simulink model "paper_Exponential_Predefined_102"  (R2019a)
settings: Solver=ode4  StartTime=0.0  StopTime=40  FixedStep=0.001  RelTol=1e-3
libraries: simulink x6
(part 2 of 3)

== matlab function paper_Exponential_Predefined_102/yuding_zhishu1 ==
  data: t input; nta_1 output; t_f input; bta1 input; bta2 input; k1 input; k2 input; p1x input; p1y input; p1z input; p2x input; p2y input; p2z input; z2x input; z2y input; z2z input; nta_2 output; nta_3 output
function [nta_1,nta_2,nta_3] = yuding(t,t_f,bta1,bta2,k1,k2,p1x,p1y,p1z,p2x,p2y,p2z,z2x,z2y,z2z)
z2x=0;
z2y=0;
z2z=0;
if 0<t & t<t_f-0.01
[nta_1,nta_2,nta_3]=im_predefined(t,t_f,bta1,bta2,k1,k2,p1x,p1y,p1z,p2x,p2y,p2z,z2x,z2y,z2z);
else 
    nta_1=0;
    nta_2=0;
    nta_3=0;
    

%     tf=t_f;
%     deta_tf=4;     
%     if tf<=t & t<(tf+deta_tf-0.01)
%         [nta_1,nta_2,nta_3]=im_predefined(t,tf+deta_tf,bta1,bta2,k1,k2,p1x,p1y,p1z,p2x,p2y,p2z,z2x,z2y,z2z); 
%     else 
%         tf=tf+deta_tf;
%         [nta_1,nta_2,nta_3]=im_predefined(t,tf+deta_tf,bta1,bta2,k1,k2,p1x,p1y,p1z,p2x,p2y,p2z,z2x,z2y,z2z); 
%     end   
%     if tf<=t & t<(tf+deta_tf-0.01)
%         [nta_1,nta_2,nta_3]=im_predefined(t,tf+deta_tf,bta1,bta2,k1,k2,p1x,p1y,p1z,p2x,p2y,p2z,z2x,z2y,z2z); 
%     else
%         tf=tf+deta_tf;
%         [nta_1,nta_2,nta_3]=im_predefined(t,tf+deta_tf,bta1,bta2,k1,k2,p1x,p1y,p1z,p2x,p2y,p2z,z2x,z2y,z2z); 
%     end  
%     if tf<=t & t<(tf+deta_tf-0.01)
%         [nta_1,nta_2,nta_3]=im_predefined(t,tf+deta_tf,bta1,bta2,k1,k2,p1x,p1y,p1z,p2x,p2y,p2z,z2x,z2y,z2z); 
%     else
%         tf=tf+deta_tf;
%         [nta_1,nta_2,nta_3]=im_predefined(t,tf+deta_tf,bta1,bta2,k1,k2,p1x,p1y,p1z,p2x,p2y,p2z,z2x,z2y,z2z); 
%     end  
%     if tf<=t & t<(tf+deta_tf-0.01)
%         [nta_1,nta_2,nta_3]=im_predefined(t,tf+deta_tf,bta1,bta2,k1,k2,p1x,p1y,p1z,p2x,p2y,p2z,z2x,z2y,z2z); 
%     else
%         tf=tf+deta_tf;
%         [nta_1,nta_2,nta_3]=im_predefined(t,tf+deta_tf,bta1,bta2,k1,k2,p1x,p1y,p1z,p2x,p2y,p2z,z2x,z2y,z2z); 
%     end  
%     if tf<=t & t<(tf+deta_tf-0.01)
%         [nta_1,nta_2,nta_3]=im_predefined(t,tf+deta_tf,bta1,bta2,k1,k2,p1x,p1y,p1z,p2x,p2y,p2z,z2x,z2y,z2z); 
%     else
%         tf=tf+deta_tf;
%         [nta_1,nta_2,nta_3]=im_predefined(t,tf+deta_tf,bta1,bta2,k1,k2,p1x,p1y,p1z,p2x,p2y,p2z,z2x,z2y,z2z); 
%     end  
%     if tf<=t & t<(tf+deta_tf-0.01)
%         [nta_1,nta_2,nta_3]=im_predefined(t,tf+deta_tf,bta1,bta2,k1,k2,p1x,p1y,p1z,p2x,p2y,p2z,z2x,z2y,z2z); 
%     else
%         tf=tf+deta_tf;
%         [nta_1,nta_2,nta_3]=im_predefined(t,tf+deta_tf,bta1,bta2,k1,k2,p1x,p1y,p1z,p2x,p2y,p2z,z2x,z2y,z2z); 
%     end  
%     if tf<=t & t<(tf+deta_tf-0.01)
%         [nta_1,nta_2,nta_3]=im_predefined(t,tf+deta_tf,bta1,bta2,k1,k2,p1x,p1y,p1z,p2x,p2y,p2z,z2x,z2y,z2z); 
%     else
%         tf=tf+deta_tf;
%         [nta_1,nta_2,nta_3]=im_predefined(t,tf+deta_tf,bta1,bta2,k1,k2,p1x,p1y,p1z,p2x,p2y,p2z,z2x,z2y,z2z); 
%     end  
%     if tf<=t & t<(tf+deta_tf)
%         [nta_1,nta_2,nta_3]=im_predefined(t,tf+deta_tf,bta1,bta2,k1,k2,p1x,p1y,p1z,p2x,p2y,p2z,z2x,z2y,z2z); 
%     else
%         tf=tf+deta_tf;
%         [nta_1,nta_2,nta_3]=im_predefined(t,tf+deta_tf,bta1,bta2,k1,k2,p1x,p1y,p1z,p2x,p2y,p2z,z2x,z2y,z2z); 
%     end  
%     if tf<=t & t<(tf+deta_tf)
%         [nta_1,nta_2,nta_3]=im_predefined(t,tf+deta_tf,bta1,bta2,k1,k2,p1x,p1y,p1z,p2x,p2y,p2z,z2x,z2y,z2z); 
%     else
%         tf=tf+deta_tf;
%         [nta_1,nta_2,nta_3]=im_predefined(t,tf+deta_tf,bta1,bta2,k1,k2,p1x,p1y,p1z,p2x,p2y,p2z,z2x,z2y,z2z); 
%     end  
%     if tf<=t & t<(tf+deta_tf)
%         [nta_1,nta_2,nta_3]=im_predefined(t,tf+deta_tf,bta1,bta2,k1,k2,p1x,p1y,p1z,p2x,p2y,p2z,z2x,z2y,z2z); 
%     else
%         tf=tf+deta_tf;
%         [nta_1,nta_2,nta_3]=im_predefined(t,tf+deta_tf,bta1,bta2,k1,k2,p1x,p1y,p1z,p2x,p2y,p2z,z2x,z2y,z2z); 
%     end  
%     if tf<=t & t<(tf+deta_tf)
%         [nta_1,nta_2,nta_3]=im_predefined(t,tf+deta_tf,bta1,bta2,k1,k2,p1x,p1y,p1z,p2x,p2y,p2z,z2x,z2y,z2z); 
%     else
%         tf=tf+deta_tf;
%         [nta_1,nta_2,nta_3]=im_predefined(t,tf+deta_tf,bta1,bta2,k1,k2,p1x,p1y,p1z,p2x,p2y,p2z,z2x,z2y,z2z); 
%     end  
%     if tf<=t & t<(tf+deta_tf)
%         [nta_1,nta_2,nta_3]=im_predefined(t,tf+deta_tf,bta1,bta2,k1,k2,p1x,p1y,p1z,p2x,p2y,p2z,z2x,z2y,z2z); 
%     else
%         tf=tf+deta_tf;
%         [nta_1,nta_2,nta_3]=im_predefined(t,tf+deta_tf,bta1,bta2,k1,k2,p1x,p1y,p1z,p2x,p2y,p2z,z2x,z2y,z2z); 
%     end  
%     if tf<=t & t<(tf+deta_tf)
%         [nta_1,nta_2,nta_3]=im_predefined(t,tf+deta_tf,bta1,bta2,k1,k2,p1x,p1y,p1z,p2x,p2y,p2z,z2x,z2y,z2z); 
%     else
%         tf=tf+deta_tf;
%         [nta_1,nta_2,nta_3]=im_predefined(t,tf+deta_tf,bta1,bta2,k1,k2,p1x,p1y,p1z,p2x,p2y,p2z,z2x,z2y,z2z); 
%     end  
%     if tf<=t & t<(tf+deta_tf)
%         [nta_1,nta_2,nta_3]=im_predefined(t,tf+deta_tf,bta1,bta2,k1,k2,p1x,p1y,p1z,p2x,p2y,p2z,z2x,z2y,z2z); 
%     else
%         tf=tf+deta_tf;
%         [nta_1,nta_2,nta_3]=im_predefined(t,tf+deta_tf,bta1,bta2,k1,k2,p1x,p1y,p1z,p2x,p2y,p2z,z2x,z2y,z2z); 
%     end  
%     if tf<=t & t<(tf+deta_tf)
%         [nta_1,nta_2,nta_3]=im_predefined(t,tf+deta_tf,bta1,bta2,k1,k2,p1x,p1y,p1z,p2x,p2y,p2z,z2x,z2y,z2z); 
%     else
%         tf=tf+deta_tf;
%         [nta_1,nta_2,nta_3]=im_predefined(t,tf+deta_tf,bta1,bta2,k1,k2,p1x,p1y,p1z,p2x,p2y,p2z,z2x,z2y,z2z); 
%     end  
%     if tf<=t & t<(tf+deta_tf)
%         [nta_1,nta_2,nta_3]=im_predefined(t,tf+deta_tf,bta1,bta2,k1,k2,p1x,p1y,p1z,p2x,p2y,p2z,z2x,z2y,z2z); 
%     else
%         tf=tf+deta_tf;
%         [nta_1,nta_2,nta_3]=im_predefined(t,tf+deta_tf,bta1,bta2,k1,k2,p1x,p1y,p1z,p2x,p2y,p2z,z2x,z2y,z2z); 
%     end  
%     if tf<=t & t<(tf+deta_tf)
%         [nta_1,nta_2,nta_3]=im_predefined(t,tf+deta_tf,bta1,bta2,k1,k2,p1x,p1y,p1z,p2x,p2y,p2z,z2x,z2y,z2z); 
%     else
%         tf=tf+deta_tf;
%         [nta_1,nta_2,nta_3]=im_predefined(t,tf+deta_tf,bta1,bta2,k1,k2,p1x,p1y,p1z,p2x,p2y,p2z,z2x,z2y,z2z); 
%     end  
%     if tf<=t & t<(tf+deta_tf)
%         [nta_1,nta_2,nta_3]=im_predefined(t,tf+deta_tf,bta1,bta2,k1,k2,p1x,p1y,p1z,p2x,p2y,p2z,z2x,z2y,z2z); 
%     else
%         tf=tf+deta_tf;
%         [nta_1,nta_2,nta_3]=im_predefined(t,tf+deta_tf,bta1,bta2,k1,k2,p1x,p1y,p1z,p2x,p2y,p2z,z2x,z2y,z2z); 
%     end  
%     if tf<=t & t<(tf+deta_tf)
%         [nta_1,nta_2,nta_3]=im_predefined(t,tf+deta_tf,bta1,bta2,k1,k2,p1x,p1y,p1z,p2x,p2y,p2z,z2x,z2y,z2z); 
%     else
%         tf=tf+deta_tf;
%         [nta_1,nta_2,nta_3]=im_predefined(t,tf+deta_tf,bta1,bta2,k1,k2,p1x,p1y,p1z,p2x,p2y,p2z,z2x,z2y,z2z); 
%     end  
%     if tf<=t & t<(tf+deta_tf)
%         [nta_1,nta_2,nta_3]=im_predefined(t,tf+deta_tf,bta1,bta2,k1,k2,p1x,p1y,p1z,p2x,p2y,p2z,z2x,z2y,z2z); 
%     else
%         tf=tf+deta_tf;
%         [nta_1,nta_2,nta_3]=im_predefined(t,tf+deta_tf,bta1,bta2,k1,k2,p1x,p1y,p1z,p2x,p2y,p2z,z2x,z2y,z2z); 
%     end  
%     if tf<=t & t<(tf+deta_tf)
%         [nta_1,nta_2,nta_3]=im_predefined(t,tf+deta_tf,bta1,bta2,k1,k2,p1x,p1y,p1z,p2x,p2y,p2z,z2x,z2y,z2z); 
%     else
%         tf=tf+deta_tf;
%         [nta_1,nta_2,nta_3]=im_predefined(t,tf+deta_tf,bta1,bta2,k1,k2,p1x,p1y,p1z,p2x,p2y,p2z,z2x,z2y,z2z); 
%     end  
%     if tf<=t & t<(tf+deta_tf)
%         [nta_1,nta_2,nta_3]=im_predefined(t,tf+deta_tf,bta1,bta2,k1,k2,p1x,p1y,p1z,p2x,p2y,p2z,z2x,z2y,z2z); 
%     else
%         tf=tf+deta_tf;
%         [nta_1,nta_2,nta_3]=im_predefined(t,tf+deta_tf,bta1,bta2,k1,k2,p1x,p1y,p1z,p2x,p2y,p2z,z2x,z2y,z2z); 
%     end  
%     if tf<=t & t<(tf+deta_tf)
%         [nta_1,nta_2,nta_3]=im_predefined(t,tf+deta_tf,bta1,bta2,k1,k2,p1x,p1y,p1z,p2x,p2y,p2z,z2x,z2y,z2z); 
%     else
%         tf=tf+deta_tf;
%         [nta_1,nta_2,nta_3]=im_predefined(t,tf+deta_tf,bta1,bta2,k1,k2,p1x,p1y,p1z,p2x,p2y,p2z,z2x,z2y,z2z); 
%     end  
%     if tf<=t & t<(tf+deta_tf)
%         [nta_1,nta_2,nta_3]=im_predefined(t,tf+deta_tf,bta1,bta2,k1,k2,p1x,p1y,p1z,p2x,p2y,p2z,z2x,z2y,z2z); 
%     else
%         tf=tf+deta_tf;
%         [nta_1,nta_2,nta_3]=im_predefined(t,tf+deta_tf,bta1,bta2,k1,k2,p1x,p1y,p1z,p2x,p2y,p2z,z2x,z2y,z2z); 
%     end  
%     if tf<=t & t<(tf+deta_tf)
%         [nta_1,nta_2,nta_3]=im_predefined(t,tf+deta_tf,bta1,bta2,k1,k2,p1x,p1y,p1z,p2x,p2y,p2z,z2x,z2y,z2z); 
%     else
%         tf=tf+deta_tf;
%         [nta_1,nta_2,nta_3]=im_predefined(t,tf+deta_tf,bta1,bta2,k1,k2,p1x,p1y,p1z,p2x,p2y,p2z,z2x,z2y,z2z); 
%     end  
%     if tf<=t & t<(tf+deta_tf)
%         [nta_1,nta_2,nta_3]=im_predefined(t,tf+deta_tf,bta1,bta2,k1,k2,p1x,p1y,p1z,p2x,p2y,p2z,z2x,z2y,z2z); 
%     else
%         tf=tf+deta_tf;
%         [nta_1,nta_2,nta_3]=im_predefined(t,tf+deta_tf,bta1,bta2,k1,k2,p1x,p1y,p1z,p2x,p2y,p2z,z2x,z2y,z2z); 
%     end  
%         if tf<=t & t<(tf+deta_tf)
%         [nta_1,nta_2,nta_3]=im_predefined(t,tf+deta_tf,bta1,bta2,k1,k2,p1x,p1y,p1z,p2x,p2y,p2z,z2x,z2y,z2z); 
%     else
%         tf=tf+deta_tf;
%         [nta_1,nta_2,nta_3]=im_predefined(t,tf+deta_tf,bta1,bta2,k1,k2,p1x,p1y,p1z,p2x,p2y,p2z,z2x,z2y,z2z); 
%     end  
%     if tf<=t & t<(tf+deta_tf)
%         [nta_1,nta_2,nta_3]=im_predefined(t,tf+deta_tf,bta1,bta2,k1,k2,p1x,p1y,p1z,p2x,p2y,p2z,z2x,z2y,z2z); 
%     else
%         tf=tf+deta_tf;
%         [nta_1,nta_2,nta_3]=im_predefined(t,tf+deta_tf,bta1,bta2,k1,k2,p1x,p1y,p1z,p2x,p2y,p2z,z2x,z2y,z2z); 
%     end  
%         if tf<=t & t<(tf+deta_tf)
%         [nta_1,nta_2,nta_3]=im_predefined(t,tf+deta_tf,bta1,bta2,k1,k2,p1x,p1y,p1z,p2x,p2y,p2z,z2x,z2y,z2z); 
%     else
%         tf=tf+deta_tf;
%         [nta_1,nta_2,nta_3]=im_predefined(t,tf+deta_tf,bta1,bta2,k1,k2,p1x,p1y,p1z,p2x,p2y,p2z,z2x,z2y,z2z); 
%     end  
%     if tf<=t & t<(tf+deta_tf)
%         [nta_1,nta_2,nta_3]=im_predefined(t,tf+deta_tf,bta1,bta2,k1,k2,p1x,p1y,p1z,p2x,p2y,p2z,z2x,z2y,z2z); 
%     else
%         tf=tf+deta_tf;
%         [nta_1,nta_2,nta_3]=im_predefined(t,tf+deta_tf,bta1,bta2,k1,k2,p1x,p1y,p1z,p2x,p2y,p2z,z2x,z2y,z2z); 
%     end  
end    
end

== matlab function paper_Exponential_Predefined_102/MATLAB Function5 ==
  data: p1y input; p2y input; z0y input; dz0y output; dz1y output; dz2y output; z1y input; z2y input
function [dz0y,dz1y,dz2y] = FTDO(p1y,p2y,z0y,z1y,z2y)
r=[24 216 864];
r0=r(1);
r1=r(2);
r2=r(3);
v0=-r0*(abs(z0y-p1y))^(0.8)*sign(z0y-p1y)-r0*(abs(z0y-p1y))^(1.2)*sign(z0y-p1y)+z1y;
dz0y=v0+p2y;
v1=-r1*(abs(z0y-p1y))^(0.6)*sign(z0y-p1y)-r1*(abs(z0y-p1y))^(1.4)*sign(z0y-p1y)+z2y;
dz1y=v1;
dz2y =-r2*(abs(z0y-p1y))^(0.4)*sign(z0y-p1y)-r2*(abs(z0y-p1y))^(1.6)*sign(z0y-p1y);
end

== matlab function paper_Exponential_Predefined_102/MATLAB Function6 ==
  data: t input; dx output; dy output; dz output; delta input; v input; gamma input; psi input
function [dx,dy,dz] = disturbance(t,delta,v,gamma,psi)
fx=-0.0005*abs(v-36)*exp((0.4*v)^0.5)+0.2*sin(psi);
fy=-0.0004*abs(v-30)*exp((0.3*v)^0.5)+0.2*cos(psi);
fz=-0.004*v^(0.5)*sin(3*gamma);
% fx=0;
% fy=0;
% fz=0;
if 0<t && t<10
    wx = 1*sin(t)+delta;
else
    wx=0;
end
if 5<t && t<15
    wy = 2*sin(2*t)-cos(3*t)+delta;
else
    wy=0;
end
if 0<t && t<20
    wz = 0.5*sin(t)+delta;
else
    wz = 0;
end

dx=fx+wx;
dy=fy+wy;
dz=fz+wz;

end

== matlab function paper_Exponential_Predefined_102/MATLAB Function7 ==
  data: p1z input; p2z input; z0z input; dz0z output; dz1z output; dz2z output; z1z input; z2z input
function [dz0z,dz1z,dz2z] = FTDO(p1z,p2z,z0z,z1z,z2z)
r=[24 216 864];
r0=r(1);
r1=r(2);
r2=r(3);
v0=-r0*(abs(z0z-p1z))^(0.8)*sign(z0z-p1z)-r0*(abs(z0z-p1z))^(1.2)*sign(z0z-p1z)+z1z;
dz0z=v0+p2z;
v1=-r1*(abs(z0z-p1z))^(0.6)*sign(z0z-p1z)-r1*(abs(z0z-p1z))^(1.4)*sign(z0z-p1z)+z2z;
dz1z=v1;
dz2z =-r2*(abs(z0z-p1z))^(0.4)*sign(z0z-p1z)-r2*(abs(z0z-p1z))^(1.6)*sign(z0z-p1z);
end

== matlab function paper_Exponential_Predefined_102/MATLAB Function8 ==
  data: p1x input; p2x input; z0x input; dz0x output; dz1x output; dz2x output; z1x input; z2x input
function [dz0x,dz1x,dz2x] = FTDO(p1x,p2x,z0x,z1x,z2x)
r=[24 216 864];%parameters of FTDO
r0=r(1);
r1=r(2);
r2=r(3);
v0=-r0*(abs(z0x-p1x))^(0.8)*sign(z0x-p1x)-r0*(abs(z0x-p1x))^(1.2)*sign(z0x-p1x)+z1x;
dz0x=v0+p2x;
v1=-r1*(abs(z0x-p1x))^(0.6)*sign(z0x-p1x)-r1*(abs(z0x-p1x))^(1.4)*sign(z0x-p1x)+z2x;
dz1x=v1;
dz2x =-r2*(abs(z0x-p1x))^(0.4)*sign(z0x-p1x)-r2*(abs(z0x-p1x))^(1.6)*sign(z0x-p1x);
end

== matlab function paper_Exponential_Predefined_102/X_dot2 ==
  data: vr input; psi_r input; gamma_r input; psi input; gamma input; v input; s1 output; s2 output; s3 output; xr_dot output; yr_dot output; zr_dot output; wx input; wy input; wz input
function [s1,s2,s3,xr_dot,yr_dot,zr_dot] = fcn(vr,psi_r,gamma_r,psi,gamma,v,wx,wy,wz)
wx=0;
wy=0;
wz=0;
s1 = v*cos(psi)*cos(gamma)+wx;
s2 = v*sin(psi)*cos(gamma)+wy;
s3 = v*sin(gamma)+wz;
xr_dot = vr*cos(psi_r)*cos(gamma_r);
yr_dot = vr*sin(psi_r)*cos(gamma_r);
zr_dot = vr*sin(gamma_r);
end

== matlab function paper_Exponential_Predefined_102/control input 2 ==
  data: a_xr input; a_yr input; a_zr input; psi input; gamma input; u1_omiga_psi output; u2_omiga_gamma output; u3_a output; v input; nta_1 input; nta_2 input; nta_3 input
function [u1_omiga_psi,u2_omiga_gamma,u3_a] = fcn(a_xr,a_yr,a_zr,psi,gamma,v,nta_1,nta_2,nta_3)
A = [-a_xr;-a_yr;-a_zr];
B = [-v*sin(psi)*cos(gamma) -v*cos(psi)*sin(gamma) cos(psi)*cos(gamma); 
    v*cos(psi)*cos(gamma) -v*sin(psi)*sin(gamma) sin(psi)*cos(gamma);
    0                        v*cos(gamma)               sin(gamma)];
nta = [nta_1 ; nta_2;nta_3];
U = -inv(B)*(A - nta);
U11=U(1,1); 
U21=U(2,1);
U31=U(3,1);
% 

u1_omiga_psi = U11 ;
u2_omiga_gamma = U21;
u3_a =U31 ;





end

== matlab function paper_Exponential_Predefined_102/f,df2 ==
  data: dx input; x input; dy input; y input; dz input; z input; dxr input; xr input; dyr input; yr input; dzr input; zr input; p1x output; p1y output; p1z output; p2x output; p2y output; p2z output; wx input; wy input; wz input; s1 output; s2 output; s3 output
 function [p1x,p1y,p1z,p2x,p2y,p2z,s1,s2,s3] = fcn(dx,x,dy,y,dz,z,dxr,xr,dyr,yr,dzr,zr,wx,wy,wz)
wx=0;
wy=0;
wz=0;
p1x = x - xr;
p1y = y - yr;
p1z = z - zr;
s1 = dx - dxr ;
s2 = dy - dyr ;
s3 = dz - dzr ;
p2x = dx - dxr-wx ;
p2y = dy - dyr-wy ;
p2z = dz - dzr-wz ;
end

== matlab function paper_Exponential_Predefined_102/u_1a1 ==
  data: u input; u_1a output
function u_1a  = fcn(u)

u_max=1;

u_1a=u_max*erf((pi^(0.5)*u)/(2*u_max));


 end

== matlab function paper_Exponential_Predefined_102/u_2a2 ==
  data: u input; u_2a output
function u_2a  = fcn(u)

u_max=1;

u_2a=u_max*erf((pi^(0.5)*u)/(2*u_max));


 end

== matlab function paper_Exponential_Predefined_102/u_3a2 ==
  data: u input; u_3a output
function u_3a  = fcn(u)

u_max=10;
v_max=15;
% u_3a=u;
u_3a=u_max*erf((pi^(0.5)*u)/(2*u_max));
% q_v=erf((pi^(0.5)*(v-25))/(2*v_max));
% % u_3a=q_u*(1-abs(q_v));
% if v>=40 & u>0
%     u_3a=0;
% elseif v<=10 & u<0
%     u_3a=0;
% else
%     u_3a=u_max*erf((pi^(0.5)*u)/(2*u_max));
    
 end

== matlab function paper_Exponential_Predefined_102/yuding_zhishu2 ==
  data: t input; nta_1 output; t_f input; bta1 input; bta2 input; k1 input; k2 input; p1x input; p1y input; p1z input; p2x input; p2y input; p2z input; z2x input; z2y input; z2z input; nta_2 output; nta_3 output
function [nta_1,nta_2,nta_3] = yuding(t,t_f,bta1,bta2,k1,k2,p1x,p1y,p1z,p2x,p2y,p2z,z2x,z2y,z2z)
z2x=0;
z2y=0;
z2z=0;
if 0<t & t<t_f-0.01
[nta_1,nta_2,nta_3]=Exponential_predefined(t,t_f,bta1,bta2,k1,k2,p1x,p1y,p1z,p2x,p2y,p2z,z2x,z2y,z2z);
else 
% tf=[]
% for i=0:1:20
% tf(i)=t_f+i;
% if tf(i)<=t &t<(tf(i)+1)
% [nta_1,nta_2,nta_3]=Exponential_predefined_yuesu(t,tf(i)+1,bta1,bta2,k1,k2,p1x,p1y,p1z,p2x,p2y,p2z,z2x,z2y,z2z);
% end
% end
    tf=t_f;
    deta_tf=4;     
    if tf<=t & t<(tf+deta_tf-0.01)
        [nta_1,nta_2,nta_3]=Exponential_predefined(t,tf+deta_tf,bta1,bta2,k1,k2,p1x,p1y,p1z,p2x,p2y,p2z,z2x,z2y,z2z); 
    else 
        tf=tf+deta_tf;
        [nta_1,nta_2,nta_3]=Exponential_predefined(t,tf+deta_tf,bta1,bta2,k1,k2,p1x,p1y,p1z,p2x,p2y,p2z,z2x,z2y,z2z); 
    end   
    if tf<=t & t<(tf+deta_tf-0.01)
        [nta_1,nta_2,nta_3]=Exponential_predefined(t,tf+deta_tf,bta1,bta2,k1,k2,p1x,p1y,p1z,p2x,p2y,p2z,z2x,z2y,z2z); 
    else
        tf=tf+deta_tf;
        [nta_1,nta_2,nta_3]=Exponential_predefined(t,tf+deta_tf,bta1,bta2,k1,k2,p1x,p1y,p1z,p2x,p2y,p2z,z2x,z2y,z2z); 
    end  
    if tf<=t & t<(tf+deta_tf-0.01)
        [nta_1,nta_2,nta_3]=Exponential_predefined(t,tf+deta_tf,bta1,bta2,k1,k2,p1x,p1y,p1z,p2x,p2y,p2z,z2x,z2y,z2z); 
    else
        tf=tf+deta_tf;
        [nta_1,nta_2,nta_3]=Exponential_predefined(t,tf+deta_tf,bta1,bta2,k1,k2,p1x,p1y,p1z,p2x,p2y,p2z,z2x,z2y,z2z); 
    end  
    if tf<=t & t<(tf+deta_tf-0.01)
        [nta_1,nta_2,nta_3]=Exponential_predefined(t,tf+deta_tf,bta1,bta2,k1,k2,p1x,p1y,p1z,p2x,p2y,p2z,z2x,z2y,z2z); 
    else
        tf=tf+deta_tf;
        [nta_1,nta_2,nta_3]=Exponential_predefined(t,tf+deta_tf,bta1,bta2,k1,k2,p1x,p1y,p1z,p2x,p2y,p2z,z2x,z2y,z2z); 
    end  
    if tf<=t & t<(tf+deta_tf-0.01)
        [nta_1,nta_2,nta_3]=Exponential_predefined(t,tf+deta_tf,bta1,bta2,k1,k2,p1x,p1y,p1z,p2x,p2y,p2z,z2x,z2y,z2z); 
    else
        tf=tf+deta_tf;
        [nta_1,nta_2,nta_3]=Exponential_predefined(t,tf+deta_tf,bta1,bta2,k1,k2,p1x,p1y,p1z,p2x,p2y,p2z,z2x,z2y,z2z); 
    end  
    if tf<=t & t<(tf+deta_tf-0.01)
        [nta_1,nta_2,nta_3]=Exponential_predefined(t,tf+deta_tf,bta1,bta2,k1,k2,p1x,p1y,p1z,p2x,p2y,p2z,z2x,z2y,z2z); 
    else
        tf=tf+deta_tf;
        [nta_1,nta_2,nta_3]=Exponential_predefined(t,tf+deta_tf,bta1,bta2,k1,k2,p1x,p1y,p1z,p2x,p2y,p2z,z2x,z2y,z2z); 
    end  
    if tf<=t & t<(tf+deta_tf-0.01)
        [nta_1,nta_2,nta_3]=Exponential_predefined(t,tf+deta_tf,bta1,bta2,k1,k2,p1x,p1y,p1z,p2x,p2y,p2z,z2x,z2y,z2z); 
    else
        tf=tf+deta_tf;
        [nta_1,nta_2,nta_3]=Exponential_predefined(t,tf+deta_tf,bta1,bta2,k1,k2,p1x,p1y,p1z,p2x,p2y,p2z,z2x,z2y,z2z); 
    end  
    if tf<=t & t<(tf+deta_tf)
        [nta_1,nta_2,nta_3]=Exponential_predefined(t,tf+deta_tf,bta1,bta2,k1,k2,p1x,p1y,p1z,p2x,p2y,p2z,z2x,z2y,z2z); 
    else
        tf=tf+deta_tf;
        [nta_1,nta_2,nta_3]=Exponential_predefined(t,tf+deta_tf,bta1,bta2,k1,k2,p1x,p1y,p1z,p2x,p2y,p2z,z2x,z2y,z2z); 
    end  
    if tf<=t & t<(tf+deta_tf)
        [nta_1,nta_2,nta_3]=Exponential_predefined(t,tf+deta_tf,bta1,bta2,k1,k2,p1x,p1y,p1z,p2x,p2y,p2z,z2x,z2y,z2z); 
    else
        tf=tf+deta_tf;
        [nta_1,nta_2,nta_3]=Exponential_predefined(t,tf+deta_tf,bta1,bta2,k1,k2,p1x,p1y,p1z,p2x,p2y,p2z,z2x,z2y,z2z); 
    end  
    if tf<=t & t<(tf+deta_tf)
        [nta_1,nta_2,nta_3]=Exponential_predefined(t,tf+deta_tf,bta1,bta2,k1,k2,p1x,p1y,p1z,p2x,p2y,p2z,z2x,z2y,z2z); 
    else
        tf=tf+deta_tf;
        [nta_1,nta_2,nta_3]=Exponential_predefined(t,tf+deta_tf,bta1,bta2,k1,k2,p1x,p1y,p1z,p2x,p2y,p2z,z2x,z2y,z2z); 
    end  
    if tf<=t & t<(tf+deta_tf)
        [nta_1,nta_2,nta_3]=Exponential_predefined(t,tf+deta_tf,bta1,bta2,k1,k2,p1x,p1y,p1z,p2x,p2y,p2z,z2x,z2y,z2z); 
    else
        tf=tf+deta_tf;
        [nta_1,nta_2,nta_3]=Exponential_predefined(t,tf+deta_tf,bta1,bta2,k1,k2,p1x,p1y,p1z,p2x,p2y,p2z,z2x,z2y,z2z); 
    end  
    if tf<=t & t<(tf+deta_tf)
        [nta_1,nta_2,nta_3]=Exponential_predefined(t,tf+deta_tf,bta1,bta2,k1,k2,p1x,p1y,p1z,p2x,p2y,p2z,z2x,z2y,z2z); 
    else
        tf=tf+deta_tf;
        [nta_1,nta_2,nta_3]=Exponential_predefined(t,tf+deta_tf,bta1,bta2,k1,k2,p1x,p1y,p1z,p2x,p2y,p2z,z2x,z2y,z2z); 
    end  
    if tf<=t & t<(tf+deta_tf)
        [nta_1,nta_2,nta_3]=Exponential_predefined(t,tf+deta_tf,bta1,bta2,k1,k2,p1x,p1y,p1z,p2x,p2y,p2z,z2x,z2y,z2z); 
    else
        tf=tf+deta_tf;
        [nta_1,nta_2,nta_3]=Exponential_predefined(t,tf+deta_tf,bta1,bta2,k1,k2,p1x,p1y,p1z,p2x,p2y,p2z,z2x,z2y,z2z); 
    end  
    if tf<=t & t<(tf+deta_tf)
        [nta_1,nta_2,nta_3]=Exponential_predefined(t,tf+deta_tf,bta1,bta2,k1,k2,p1x,p1y,p1z,p2x,p2y,p2z,z2x,z2y,z2z); 
    else
        tf=tf+deta_tf;
        [nta_1,nta_2,nta_3]=Exponential_predefined(t,tf+deta_tf,bta1,bta2,k1,k2,p1x,p1y,p1z,p2x,p2y,p2z,z2x,z2y,z2z); 
    end  
    if tf<=t & t<(tf+deta_tf)
        [nta_1,nta_2,nta_3]=Exponential_predefined(t,tf+deta_tf,bta1,bta2,k1,k2,p1x,p1y,p1z,p2x,p2y,p2z,z2x,z2y,z2z); 
    else
        tf=tf+deta_tf;
        [nta_1,nta_2,nta_3]=Exponential_predefined(t,tf+deta_tf,bta1,bta2,k1,k2,p1x,p1y,p1z,p2x,p2y,p2z,z2x,z2y,z2z); 
    end  
    if tf<=t & t<(tf+deta_tf)
        [nta_1,nta_2,nta_3]=Exponential_predefined(t,tf+deta_tf,bta1,bta2,k1,k2,p1x,p1y,p1z,p2x,p2y,p2z,z2x,z2y,z2z); 
    else
        tf=tf+deta_tf;
        [nta_1,nta_2,nta_3]=Exponential_predefined(t,tf+deta_tf,bta1,bta2,k1,k2,p1x,p1y,p1z,p2x,p2y,p2z,z2x,z2y,z2z); 
    end  
    if tf<=t & t<(tf+deta_tf)
        [nta_1,nta_2,nta_3]=Exponential_predefined(t,tf+deta_tf,bta1,bta2,k1,k2,p1x,p1y,p1z,p2x,p2y,p2z,z2x,z2y,z2z); 
    else
        tf=tf+deta_tf;
        [nta_1,nta_2,nta_3]=Exponential_predefined(t,tf+deta_tf,bta1,bta2,k1,k2,p1x,p1y,p1z,p2x,p2y,p2z,z2x,z2y,z2z); 
    end  
    if tf<=t & t<(tf+deta_tf)
        [nta_1,nta_2,nta_3]=Exponential_predefined(t,tf+deta_tf,bta1,bta2,k1,k2,p1x,p1y,p1z,p2x,p2y,p2z,z2x,z2y,z2z); 
    else
        tf=tf+deta_tf;
        [nta_1,nta_2,nta_3]=Exponential_predefined(t,tf+deta_tf,bta1,bta2,k1,k2,p1x,p1y,p1z,p2x,p2y,p2z,z2x,z2y,z2z); 
    end  
    if tf<=t & t<(tf+deta_tf)
        [nta_1,nta_2,nta_3]=Exponential_predefined(t,tf+deta_tf,bta1,bta2,k1,k2,p1x,p1y,p1z,p2x,p2y,p2z,z2x,z2y,z2z); 
    else
        tf=tf+deta_tf;
        [nta_1,nta_2,nta_3]=Exponential_predefined(t,tf+deta_tf,bta1,bta2,k1,k2,p1x,p1y,p1z,p2x,p2y,p2z,z2x,z2y,z2z); 
    end  
    if tf<=t & t<(tf+deta_tf)
        [nta_1,nta_2,nta_3]=Exponential_predefined(t,tf+deta_tf,bta1,bta2,k1,k2,p1x,p1y,p1z,p2x,p2y,p2z,z2x,z2y,z2z); 
    else
        tf=tf+deta_tf;
        [nta_1,nta_2,nta_3]=Exponential_predefined(t,tf+deta_tf,bta1,bta2,k1,k2,p1x,p1y,p1z,p2x,p2y,p2z,z2x,z2y,z2z); 
    end  
    if tf<=t & t<(tf+deta_tf)
        [nta_1,nta_2,nta_3]=Exponential_predefined(t,tf+deta_tf,bta1,bta2,k1,k2,p1x,p1y,p1z,p2x,p2y,p2z,z2x,z2y,z2z); 
    else
        tf=tf+deta_tf;
        [nta_1,nta_2,nta_3]=Exponential_predefined(t,tf+deta_tf,bta1,bta2,k1,k2,p1x,p1y,p1z,p2x,p2y,p2z,z2x,z2y,z2z); 
    end  
    if tf<=t & t<(tf+deta_tf)
        [nta_1,nta_2,nta_3]=Exponential_predefined(t,tf+deta_tf,bta1,bta2,k1,k2,p1x,p1y,p1z,p2x,p2y,p2z,z2x,z2y,z2z); 
    else
        tf=tf+deta_tf;
        [nta_1,nta_2,nta_3]=Exponential_predefined(t,tf+deta_tf,bta1,bta2,k1,k2,p1x,p1y,p1z,p2x,p2y,p2z,z2x,z2y,z2z); 
    end  
    if tf<=t & t<(tf+deta_tf)
        [nta_1,nta_2,nta_3]=Exponential_predefined(t,tf+deta_tf,bta1,bta2,k1,k2,p1x,p1y,p1z,p2x,p2y,p2z,z2x,z2y,z2z); 
    else
        tf=tf+deta_tf;
        [nta_1,nta_2,nta_3]=Exponential_predefined(t,tf+deta_tf,bta1,bta2,k1,k2,p1x,p1y,p1z,p2x,p2y,p2z,z2x,z2y,z2z); 
    end  
    if tf<=t & t<(tf+deta_tf)
        [nta_1,nta_2,nta_3]=Exponential_predefined(t,tf+deta_tf,bta1,bta2,k1,k2,p1x,p1y,p1z,p2x,p2y,p2z,z2x,z2y,z2z); 
    else
        tf=tf+deta_tf;
        [nta_1,nta_2,nta_3]=Exponential_predefined(t,tf+deta_tf,bta1,bta2,k1,k2,p1x,p1y,p1z,p2x,p2y,p2z,z2x,z2y,z2z); 
    end  
    if tf<=t & t<(tf+deta_tf)
        [nta_1,nta_2,nta_3]=Exponential_predefined(t,tf+deta_tf,bta1,bta2,k1,k2,p1x,p1y,p1z,p2x,p2y,p2z,z2x,z2y,z2z); 
    else
        tf=tf+deta_tf;
        [nta_1,nta_2,nta_3]=Exponential_predefined(t,tf+deta_tf,bta1,bta2,k1,k2,p1x,p1y,p1z,p2x,p2y,p2z,z2x,z2y,z2z); 
    end  
    if tf<=t & t<(tf+deta_tf)
        [nta_1,nta_2,nta_3]=Exponential_predefined(t,tf+deta_tf,bta1,bta2,k1,k2,p1x,p1y,p1z,p2x,p2y,p2z,z2x,z2y,z2z); 
    else
        tf=tf+deta_tf;
        [nta_1,nta_2,nta_3]=Exponential_predefined(t,tf+deta_tf,bta1,bta2,k1,k2,p1x,p1y,p1z,p2x,p2y,p2z,z2x,z2y,z2z); 
    end  
        if tf<=t & t<(tf+deta_tf)
        [nta_1,nta_2,nta_3]=Exponential_predefined(t,tf+deta_tf,bta1,bta2,k1,k2,p1x,p1y,p1z,p2x,p2y,p2z,z2x,z2y,z2z); 
    else
        tf=tf+deta_tf;
        [nta_1,nta_2,nta_3]=Exponential_predefined(t,tf+deta_tf,bta1,bta2,k1,k2,p1x,p1y,p1z,p2x,p2y,p2z,z2x,z2y,z2z); 
    end  
    if tf<=t & t<(tf+deta_tf)
        [nta_1,nta_2,nta_3]=Exponential_predefined(t,tf+deta_tf,bta1,bta2,k1,k2,p1x,p1y,p1z,p2x,p2y,p2z,z2x,z2y,z2z); 
    else
        tf=tf+deta_tf;
        [nta_1,nta_2,nta_3]=Exponential_predefined(t,tf+deta_tf,bta1,bta2,k1,k2,p1x,p1y,p1z,p2x,p2y,p2z,z2x,z2y,z2z); 
    end  
        if tf<=t & t<(tf+deta_tf)
        [nta_1,nta_2,nta_3]=Exponential_predefined(t,tf+deta_tf,bta1,bta2,k1,k2,p1x,p1y,p1z,p2x,p2y,p2z,z2x,z2y,z2z); 
    else
        tf=tf+deta_tf;
        [nta_1,nta_2,nta_3]=Exponential_predefined(t,tf+deta_tf,bta1,bta2,k1,k2,p1x,p1y,p1z,p2x,p2y,p2z,z2x,z2y,z2z); 
    end  
    if tf<=t & t<(tf+deta_tf)
        [nta_1,nta_2,nta_3]=Exponential_predefined(t,tf+deta_tf,bta1,bta2,k1,k2,p1x,p1y,p1z,p2x,p2y,p2z,z2x,z2y,z2z); 
    else
        tf=tf+deta_tf;
        [nta_1,nta_2,nta_3]=Exponential_predefined(t,tf+deta_tf,bta1,bta2,k1,k2,p1x,p1y,p1z,p2x,p2y,p2z,z2x,z2y,z2z); 
    end  
end    
end

== matlab function paper_Exponential_Predefined_102/ a^r3 ==
  data: ar input; vr input; a_xr output; a_yr output; omiga_psi_r input; psi_r input; omiga_gamma_r input; a_zr output; gamma_r input
function [a_xr,a_yr,a_zr] = fcn(ar,vr,omiga_psi_r,psi_r,omiga_gamma_r,gamma_r)
a_xr = -vr*sin(psi_r)*cos(gamma_r)*omiga_psi_r-vr*cos(psi_r)*sin(gamma_r)*omiga_gamma_r+cos(psi_r)*cos(gamma_r)*ar;
a_yr = vr*cos(psi_r)*cos(gamma_r)*omiga_psi_r-vr*sin(psi_r)*sin(gamma_r)*omiga_gamma_r+ sin(psi_r)*cos(gamma_r)*ar;
a_zr = vr*cos(gamma_r)*omiga_gamma_r + sin(gamma_r)*ar;
end

== matlab function paper_Exponential_Predefined_102/MATLAB Function10 ==
  data: t input; dx output; dy output; dz output; delta input; v input; gamma input; psi input
function [dx,dy,dz] = disturbance(t,delta,v,gamma,psi)
fx=-0.0005*abs(v-36)*exp((0.4*v)^0.5)+0.2*sin(psi);
fy=-0.0004*abs(v-30)*exp((0.3*v)^0.5)+0.2*cos(psi);
fz=-0.004*v^(0.5)*sin(3*gamma);
% fx=0;
% fy=0;
% fz=0;
if 0<t && t<10
    wx = 1*sin(t)+delta;
else
    wx=0;
end
if 5<t && t<15
    wy = 2*sin(2*t)-cos(3*t)+delta;
else
    wy=0;
end
if 0<t && t<20
    wz = 0.5*sin(t)+delta;
else
    wz = 0;
end

dx=fx+wx;
dy=fy+wy;
dz=fz+wz;

end

== matlab function paper_Exponential_Predefined_102/MATLAB Function11 ==
  data: p1z input; p2z input; z0z input; dz0z output; dz1z output; dz2z output; z1z input; z2z input
function [dz0z,dz1z,dz2z] = FTDO(p1z,p2z,z0z,z1z,z2z)
r=[24 216 864];
r0=r(1);
r1=r(2);
r2=r(3);
v0=-r0*(abs(z0z-p1z))^(0.8)*sign(z0z-p1z)-r0*(abs(z0z-p1z))^(1.2)*sign(z0z-p1z)+z1z;
dz0z=v0+p2z;
v1=-r1*(abs(z0z-p1z))^(0.6)*sign(z0z-p1z)-r1*(abs(z0z-p1z))^(1.4)*sign(z0z-p1z)+z2z;
dz1z=v1;
dz2z =-r2*(abs(z0z-p1z))^(0.4)*sign(z0z-p1z)-r2*(abs(z0z-p1z))^(1.6)*sign(z0z-p1z);
end

== matlab function paper_Exponential_Predefined_102/MATLAB Function12 ==
  data: p1x input; p2x input; z0x input; dz0x output; dz1x output; dz2x output; z1x input; z2x input
function [dz0x,dz1x,dz2x] = FTDO(p1x,p2x,z0x,z1x,z2x)
r=[24 216 864];
r0=r(1);
r1=r(2);
r2=r(3);
v0=-r0*(abs(z0x-p1x))^(0.8)*sign(z0x-p1x)-r0*(abs(z0x-p1x))^(1.2)*sign(z0x-p1x)+z1x;
dz0x=v0+p2x;
% dz0x=v0;
v1=-r1*(abs(z0x-p1x))^(0.6)*sign(z0x-p1x)-r1*(abs(z0x-p1x))^(1.4)*sign(z0x-p1x)+z2x;
dz1x=v1;
dz2x =-r2*(abs(z0x-p1x))^(0.4)*sign(z0x-p1x)-r2*(abs(z0x-p1x))^(1.6)*sign(z0x-p1x);
end

== matlab function paper_Exponential_Predefined_102/MATLAB Function9 ==
  data: p1y input; p2y input; z0y input; dz0y output; dz1y output; dz2y output; z1y input; z2y input
function [dz0y,dz1y,dz2y] = FTDO(p1y,p2y,z0y,z1y,z2y)
r=[24 216 864];
r0=r(1);
r1=r(2);
r2=r(3);
v0=-r0*(abs(z0y-p1y))^(0.8)*sign(z0y-p1y)-r0*(abs(z0y-p1y))^(1.2)*sign(z0y-p1y)+z1y;
dz0y=v0+p2y;
v1=-r1*(abs(z0y-p1y))^(0.6)*sign(z0y-p1y)-r1*(abs(z0y-p1y))^(1.4)*sign(z0y-p1y)+z2y;
dz1y=v1;
dz2y =-r2*(abs(z0y-p1y))^(0.4)*sign(z0y-p1y)-r2*(abs(z0y-p1y))^(1.6)*sign(z0y-p1y);
end

== matlab function paper_Exponential_Predefined_102/X_dot3 ==
  data: vr input; psi_r input; gamma_r input; psi input; gamma input; v input; s1 output; s2 output; s3 output; xr_dot output; yr_dot output; zr_dot output; wx input; wy input; wz input
function [s1,s2,s3,xr_dot,yr_dot,zr_dot] = fcn(vr,psi_r,gamma_r,psi,gamma,v,wx,wy,wz)
% wx=0;
% wy=0;
% wz=0;
s1 = v*cos(psi)*cos(gamma)+wx;
s2 = v*sin(psi)*cos(gamma)+wy;
s3 = v*sin(gamma)+wz;
xr_dot = vr*cos(psi_r)*cos(gamma_r);
yr_dot = vr*sin(psi_r)*cos(gamma_r);
zr_dot = vr*sin(gamma_r);
end

== matlab function paper_Exponential_Predefined_102/control input 3 ==
  data: a_xr input; a_yr input; a_zr input; psi input; gamma input; u1_omiga_psi output; u2_omiga_gamma output; u3_a output; v input; nta_1 input; nta_2 input; nta_3 input
function [u1_omiga_psi,u2_omiga_gamma,u3_a] = fcn(a_xr,a_yr,a_zr,psi,gamma,v,nta_1,nta_2,nta_3)
A = [-a_xr;-a_yr;-a_zr];
B = [-v*sin(psi)*cos(gamma) -v*cos(psi)*sin(gamma) cos(psi)*cos(gamma); 
    v*cos(psi)*cos(gamma) -v*sin(psi)*sin(gamma) sin(psi)*cos(gamma);
    0                        v*cos(gamma)               sin(gamma)];
nta = [nta_1 ; nta_2;nta_3];
U = -inv(B)*(A - nta);
U11=U(1,1); 
U21=U(2,1);
U31=U(3,1);
% 

u1_omiga_psi = U11 ;
u2_omiga_gamma = U21;
u3_a =U31 ;
%%添加约束





end

== matlab function paper_Exponential_Predefined_102/f,df3 ==
  data: dx input; x input; dy input; y input; dz input; z input; dxr input; xr input; dyr input; yr input; dzr input; zr input; p1x output; p1y output; p1z output; p2x output; p2y output; p2z output; wx input; wy input; wz input; s1 output; s2 output; s3 output
 function [p1x,p1y,p1z,p2x,p2y,p2z,s1,s2,s3] = fcn(dx,x,dy,y,dz,z,dxr,xr,dyr,yr,dzr,zr,wx,wy,wz)
% wx=0;
% wy=0;
% wz=0;
p1x = x - xr;
p1y = y - yr;
p1z = z - zr;
s1 = dx - dxr ;
s2 = dy - dyr ;
s3 = dz - dzr ;
p2x = dx - dxr-wx ;
p2y = dy - dyr-wy ;
p2z = dz - dzr-wz ;
end

== matlab function paper_Exponential_Predefined_102/u_1a3 ==
  data: u input; u_1a output
function u_1a  = fcn(u)

u_max=1.6;

u_1a=u_max*erf((pi^(0.5)*u)/(2*u_max));


 end

== matlab function paper_Exponential_Predefined_102/u_2a3 ==
  data: u input; u_2a output
function u_2a  = fcn(u)

u_max=1.6;

u_2a=u_max*erf((pi^(0.5)*u)/(2*u_max));


 end

== matlab function paper_Exponential_Predefined_102/u_3a3 ==
  data: u input; u_3a output
function u_3a  = fcn(u)

u_max=17;
v_max=15;
% u_3a=u;
u_3a=u_max*erf((pi^(0.5)*u)/(2*u_max));
% q_v=erf((pi^(0.5)*(v-25))/(2*v_max));
% % u_3a=q_u*(1-abs(q_v));
% if v>=40 & u>0
%     u_3a=0;
% elseif v<=10 & u<0
%     u_3a=0;
% else
%     u_3a=u_max*erf((pi^(0.5)*u)/(2*u_max));
    
 end

== matlab function paper_Exponential_Predefined_102/yuding_zhishu3 ==
  data: t input; nta_1 output; t_f input; bta1 input; bta2 input; k1 input; k2 input; p1x input; p1y input; p1z input; p2x input; p2y input; p2z input; z2x input; z2y input; z2z input; nta_2 output; nta_3 output
function [nta_1,nta_2,nta_3] = predefined(t,t_f,bta1,bta2,k1,k2,p1x,p1y,p1z,p2x,p2y,p2z,z2x,z2y,z2z)
% z2x=0;
% z2y=0;
% z2z=0;
if 0<t & t<t_f-0.01
[nta_1,nta_2,nta_3]=im_predefined(t,t_f,bta1,bta2,k1,k2,p1x,p1y,p1z,p2x,p2y,p2z,z2x,z2y,z2z);
else 
%     nta_1=0;
%     nta_2=0;       
%     nta_3=0;
    

    tf=t_f;
    deta_tf=10;     
    if tf<=t & t<(tf+deta_tf-0.01)
        [nta_1,nta_2,nta_3]=im_predefined(t,tf+deta_tf,bta1,bta2,k1,k2,p1x,p1y,p1z,p2x,p2y,p2z,z2x,z2y,z2z); 
    else 
        tf=tf+deta_tf;
        [nta_1,nta_2,nta_3]=im_predefined(t,tf+deta_tf,bta1,bta2,k1,k2,p1x,p1y,p1z,p2x,p2y,p2z,z2x,z2y,z2z); 
    end   
    if tf<=t & t<(tf+deta_tf-0.01)
        [nta_1,nta_2,nta_3]=im_predefined(t,tf+deta_tf,bta1,bta2,k1,k2,p1x,p1y,p1z,p2x,p2y,p2z,z2x,z2y,z2z); 
    else
        tf=tf+deta_tf;
        [nta_1,nta_2,nta_3]=im_predefined(t,tf+deta_tf,bta1,bta2,k1,k2,p1x,p1y,p1z,p2x,p2y,p2z,z2x,z2y,z2z); 
    end  
    if tf<=t & t<(tf+deta_tf-0.01)
        [nta_1,nta_2,nta_3]=im_predefined(t,tf+deta_tf,bta1,bta2,k1,k2,p1x,p1y,p1z,p2x,p2y,p2z,z2x,z2y,z2z); 
    else
        tf=tf+deta_tf;
        [nta_1,nta_2,nta_3]=im_predefined(t,tf+deta_tf,bta1,bta2,k1,k2,p1x,p1y,p1z,p2x,p2y,p2z,z2x,z2y,z2z); 
    end  
    if tf<=t & t<(tf+deta_tf-0.01)
        [nta_1,nta_2,nta_3]=im_predefined(t,tf+deta_tf,bta1,bta2,k1,k2,p1x,p1y,p1z,p2x,p2y,p2z,z2x,z2y,z2z); 
    else
        tf=tf+deta_tf;
        [nta_1,nta_2,nta_3]=im_predefined(t,tf+deta_tf,bta1,bta2,k1,k2,p1x,p1y,p1z,p2x,p2y,p2z,z2x,z2y,z2z); 
    end  
    if tf<=t & t<(tf+deta_tf-0.01)
        [nta_1,nta_2,nta_3]=im_predefined(t,tf+deta_tf,bta1,bta2,k1,k2,p1x,p1y,p1z,p2x,p2y,p2z,z2x,z2y,z2z); 
    else
        tf=tf+deta_tf;
        [nta_1,nta_2,nta_3]=im_predefined(t,tf+deta_tf,bta1,bta2,k1,k2,p1x,p1y,p1z,p2x,p2y,p2z,z2x,z2y,z2z); 
    end  
    if tf<=t & t<(tf+deta_tf-0.01)
        [nta_1,nta_2,nta_3]=im_predefined(t,tf+deta_tf,bta1,bta2,k1,k2,p1x,p1y,p1z,p2x,p2y,p2z,z2x,z2y,z2z); 
    else
        tf=tf+deta_tf;
        [nta_1,nta_2,nta_3]=im_predefined(t,tf+deta_tf,bta1,bta2,k1,k2,p1x,p1y,p1z,p2x,p2y,p2z,z2x,z2y,z2z); 
    end  
    if tf<=t & t<(tf+deta_tf-0.01)
        [nta_1,nta_2,nta_3]=im_predefined(t,tf+deta_tf,bta1,bta2,k1,k2,p1x,p1y,p1z,p2x,p2y,p2z,z2x,z2y,z2z); 
    else
        tf=tf+deta_tf;
        [nta_1,nta_2,nta_3]=im_predefined(t,tf+deta_tf,bta1,bta2,k1,k2,p1x,p1y,p1z,p2x,p2y,p2z,z2x,z2y,z2z); 
    end  
    if tf<=t & t<(tf+deta_tf)
        [nta_1,nta_2,nta_3]=im_predefined(t,tf+deta_tf,bta1,bta2,k1,k2,p1x,p1y,p1z,p2x,p2y,p2z,z2x,z2y,z2z); 
    else
        tf=tf+deta_tf;
        [nta_1,nta_2,nta_3]=im_predefined(t,tf+deta_tf,bta1,bta2,k1,k2,p1x,p1y,p1z,p2x,p2y,p2z,z2x,z2y,z2z); 
    end  
    if tf<=t & t<(tf+deta_tf)
        [nta_1,nta_2,nta_3]=im_predefined(t,tf+deta_tf,bta1,bta2,k1,k2,p1x,p1y,p1z,p2x,p2y,p2z,z2x,z2y,z2z); 
    else
        tf=tf+deta_tf;
        [nta_1,nta_2,nta_3]=im_predefined(t,tf+deta_tf,bta1,bta2,k1,k2,p1x,p1y,p1z,p2x,p2y,p2z,z2x,z2y,z2z); 
    end  
    if tf<=t & t<(tf+deta_tf)
        [nta_1,nta_2,nta_3]=im_predefined(t,tf+deta_tf,bta1,bta2,k1,k2,p1x,p1y,p1z,p2x,p2y,p2z,z2x,z2y,z2z); 
    else
        tf=tf+deta_tf;
        [nta_1,nta_2,nta_3]=im_predefined(t,tf+deta_tf,bta1,bta2,k1,k2,p1x,p1y,p1z,p2x,p2y,p2z,z2x,z2y,z2z); 
    end  
    if tf<=t & t<(tf+deta_tf)
        [nta_1,nta_2,nta_3]=im_predefined(t,tf+deta_tf,bta1,bta2,k1,k2,p1x,p1y,p1z,p2x,p2y,p2z,z2x,z2y,z2z); 
    else
        tf=tf+deta_tf;
        [nta_1,nta_2,nta_3]=im_predefined(t,tf+deta_tf,bta1,bta2,k1,k2,p1x,p1y,p1z,p2x,p2y,p2z,z2x,z2y,z2z); 
    end  
    if tf<=t & t<(tf+deta_tf)
        [nta_1,nta_2,nta_3]=im_predefined(t,tf+deta_tf,bta1,bta2,k1,k2,p1x,p1y,p1z,p2x,p2y,p2z,z2x,z2y,z2z); 
    else
        tf=tf+deta_tf;
        [nta_1,nta_2,nta_3]=im_predefined(t,tf+deta_tf,bta1,bta2,k1,k2,p1x,p1y,p1z,p2x,p2y,p2z,z2x,z2y,z2z); 
    end  
    if tf<=t & t<(tf+deta_tf)
        [nta_1,nta_2,nta_3]=im_predefined(t,tf+deta_tf,bta1,bta2,k1,k2,p1x,p1y,p1z,p2x,p2y,p2z,z2x,z2y,z2z); 
    else
        tf=tf+deta_tf;
        [nta_1,nta_2,nta_3]=im_predefined(t,tf+deta_tf,bta1,bta2,k1,k2,p1x,p1y,p1z,p2x,p2y,p2z,z2x,z2y,z2z); 
    end  
    if tf<=t & t<(tf+deta_tf)
        [nta_1,nta_2,nta_3]=im_predefined(t,tf+deta_tf,bta1,bta2,k1,k2,p1x,p1y,p1z,p2x,p2y,p2z,z2x,z2y,z2z); 
    else
        tf=tf+deta_tf;
        [nta_1,nta_2,nta_3]=im_predefined(t,tf+deta_tf,bta1,bta2,k1,k2,p1x,p1y,p1z,p2x,p2y,p2z,z2x,z2y,z2z); 
    end  
    if tf<=t & t<(tf+deta_tf)
        [nta_1,nta_2,nta_3]=im_predefined(t,tf+deta_tf,bta1,bta2,k1,k2,p1x,p1y,p1z,p2x,p2y,p2z,z2x,z2y,z2z); 
    else
        tf=tf+deta_tf;
        [nta_1,nta_2,nta_3]=im_predefined(t,tf+deta_tf,bta1,bta2,k1,k2,p1x,p1y,p1z,p2x,p2y,p2z,z2x,z2y,z2z); 
    end  
    if tf<=t & t<(tf+deta_tf)
        [nta_1,nta_2,nta_3]=im_predefined(t,tf+deta_tf,bta1,bta2,k1,k2,p1x,p1y,p1z,p2x,p2y,p2z,z2x,z2y,z2z); 
    else
        tf=tf+deta_tf;
        [nta_1,nta_2,nta_3]=im_predefined(t,tf+deta_tf,bta1,bta2,k1,k2,p1x,p1y,p1z,p2x,p2y,p2z,z2x,z2y,z2z); 
    end  
    if tf<=t & t<(tf+deta_tf)
        [nta_1,nta_2,nta_3]=im_predefined(t,tf+deta_tf,bta1,bta2,k1,k2,p1x,p1y,p1z,p2x,p2y,p2z,z2x,z2y,z2z); 
    else
        tf=tf+deta_tf;
        [nta_1,nta_2,nta_3]=im_predefined(t,tf+deta_tf,bta1,bta2,k1,k2,p1x,p1y,p1z,p2x,p2y,p2z,z2x,z2y,z2z); 
    end  
    if tf<=t & t<(tf+deta_tf)
        [nta_1,nta_2,nta_3]=im_predefined(t,tf+deta_tf,bta1,bta2,k1,k2,p1x,p1y,p1z,p2x,p2y,p2z,z2x,z2y,z2z); 
    else
        tf=tf+deta_tf;
        [nta_1,nta_2,nta_3]=im_predefined(t,tf+deta_tf,bta1,bta2,k1,k2,p1x,p1y,p1z,p2x,p2y,p2z,z2x,z2y,z2z); 
    end  
    if tf<=t & t<(tf+deta_tf)
        [nta_1,nta_2,nta_3]=im_predefined(t,tf+deta_tf,bta1,bta2,k1,k2,p1x,p1y,p1z,p2x,p2y,p2z,z2x,z2y,z2z); 
    else
        tf=tf+deta_tf;
        [nta_1,nta_2,nta_3]=im_predefined(t,tf+deta_tf,bta1,bta2,k1,k2,p1x,p1y,p1z,p2x,p2y,p2z,z2x,z2y,z2z); 
    end  
    if tf<=t & t<(tf+deta_tf)
        [nta_1,nta_2,nta_3]=im_predefined(t,tf+deta_tf,bta1,bta2,k1,k2,p1x,p1y,p1z,p2x,p2y,p2z,z2x,z2y,z2z); 
    else
        tf=tf+deta_tf;
        [nta_1,nta_2,nta_3]=im_predefined(t,tf+deta_tf,bta1,bta2,k1,k2,p1x,p1y,p1z,p2x,p2y,p2z,z2x,z2y,z2z); 
    end  
    if tf<=t & t<(tf+deta_tf)
        [nta_1,nta_2,nta_3]=im_predefined(t,tf+deta_tf,bta1,bta2,k1,k2,p1x,p1y,p1z,p2x,p2y,p2z,z2x,z2y,z2z); 
    else
        tf=tf+deta_tf;
        [nta_1,nta_2,nta_3]=im_predefined(t,tf+deta_tf,bta1,bta2,k1,k2,p1x,p1y,p1z,p2x,p2y,p2z,z2x,z2y,z2z); 
    end  
    if tf<=t & t<(tf+deta_tf)
        [nta_1,nta_2,nta_3]=im_predefined(t,tf+deta_tf,bta1,bta2,k1,k2,p1x,p1y,p1z,p2x,p2y,p2z,z2x,z2y,z2z); 
    else
        tf=tf+deta_tf;
        [nta_1,nta_2,nta_3]=im_predefined(t,tf+deta_tf,bta1,bta2,k1,k2,p1x,p1y,p1z,p2x,p2y,p2z,z2x,z2y,z2z); 
    end  
    if tf<=t & t<(tf+deta_tf)
        [nta_1,nta_2,nta_3]=im_predefined(t,tf+deta_tf,bta1,bta2,k1,k2,p1x,p1y,p1z,p2x,p2y,p2z,z2x,z2y,z2z); 
    else
        tf=tf+deta_tf;
        [nta_1,nta_2,nta_3]=im_predefined(t,tf+deta_tf,bta1,bta2,k1,k2,p1x,p1y,p1z,p2x,p2y,p2z,z2x,z2y,z2z); 
    end  
    if tf<=t & t<(tf+deta_tf)
        [nta_1,nta_2,nta_3]=im_predefined(t,tf+deta_tf,bta1,bta2,k1,k2,p1x,p1y,p1z,p2x,p2y,p2z,z2x,z2y,z2z); 
    else
        tf=tf+deta_tf;
        [nta_1,nta_2,nta_3]=im_predefined(t,tf+deta_tf,bta1,bta2,k1,k2,p1x,p1y,p1z,p2x,p2y,p2z,z2x,z2y,z2z); 
    end  
    if tf<=t & t<(tf+deta_tf)
        [nta_1,nta_2,nta_3]=im_predefined(t,tf+deta_tf,bta1,bta2,k1,k2,p1x,p1y,p1z,p2x,p2y,p2z,z2x,z2y,z2z); 
    else
        tf=tf+deta_tf;
        [nta_1,nta_2,nta_3]=im_predefined(t,tf+deta_tf,bta1,bta2,k1,k2,p1x,p1y,p1z,p2x,p2y,p2z,z2x,z2y,z2z); 
    end  
    if tf<=t & t<(tf+deta_tf)
        [nta_1,nta_2,nta_3]=im_predefined(t,tf+deta_tf,bta1,bta2,k1,k2,p1x,p1y,p1z,p2x,p2y,p2z,z2x,z2y,z2z); 
    else
        tf=tf+deta_tf;
        [nta_1,nta_2,nta_3]=im_predefined(t,tf+deta_tf,bta1,bta2,k1,k2,p1x,p1y,p1z,p2x,p2y,p2z,z2x,z2y,z2z); 
    end  
        if tf<=t & t<(tf+deta_tf)
        [nta_1,nta_2,nta_3]=im_predefined(t,tf+deta_tf,bta1,bta2,k1,k2,p1x,p1y,p1z,p2x,p2y,p2z,z2x,z2y,z2z); 
    else
        tf=tf+deta_tf;
        [nta_1,nta_2,nta_3]=im_predefined(t,tf+deta_tf,bta1,bta2,k1,k2,p1x,p1y,p1z,p2x,p2y,p2z,z2x,z2y,z2z); 
    end  
    if tf<=t & t<(tf+deta_tf)
        [nta_1,nta_2,nta_3]=im_predefined(t,tf+deta_tf,bta1,bta2,k1,k2,p1x,p1y,p1z,p2x,p2y,p2z,z2x,z2y,z2z); 
    else
        tf=tf+deta_tf;
        [nta_1,nta_2,nta_3]=im_predefined(t,tf+deta_tf,bta1,bta2,k1,k2,p1x,p1y,p1z,p2x,p2y,p2z,z2x,z2y,z2z); 
    end  
        if tf<=t & t<(tf+deta_tf)
        [nta_1,nta_2,nta_3]=im_predefined(t,tf+deta_tf,bta1,bta2,k1,k2,p1x,p1y,p1z,p2x,p2y,p2z,z2x,z2y,z2z); 
    else
        tf=tf+deta_tf;
        [nta_1,nta_2,nta_3]=im_predefined(t,tf+deta_tf,bta1,bta2,k1,k2,p1x,p1y,p1z,p2x,p2y,p2z,z2x,z2y,z2z); 
    end  
    if tf<=t & t<(tf+deta_tf)
        [nta_1,nta_2,nta_3]=im_predefined(t,tf+deta_tf,bta1,bta2,k1,k2,p1x,p1y,p1z,p2x,p2y,p2z,z2x,z2y,z2z); 
    else
        tf=tf+deta_tf;
        [nta_1,nta_2,nta_3]=im_predefined(t,tf+deta_tf,bta1,bta2,k1,k2,p1x,p1y,p1z,p2x,p2y,p2z,z2x,z2y,z2z); 
    end  
end    
end

== matlab function paper_Exponential_Predefined_102/ a^r4 ==
  data: ar input; vr input; a_xr output; a_yr output; omiga_psi_r input; psi_r input; omiga_gamma_r input; a_zr output; gamma_r input
function [a_xr,a_yr,a_zr] = fcn(ar,vr,omiga_psi_r,psi_r,omiga_gamma_r,gamma_r)
a_xr = -vr*sin(psi_r)*cos(gamma_r)*omiga_psi_r-vr*cos(psi_r)*sin(gamma_r)*omiga_gamma_r+cos(psi_r)*cos(gamma_r)*ar;
a_yr = vr*cos(psi_r)*cos(gamma_r)*omiga_psi_r-vr*sin(psi_r)*sin(gamma_r)*omiga_gamma_r+ sin(psi_r)*cos(gamma_r)*ar;
a_zr = vr*cos(gamma_r)*omiga_gamma_r + sin(gamma_r)*ar;
end

== matlab function paper_Exponential_Predefined_102/MATLAB Function13 ==
  data: p1y input; p2y input; z0y input; dz0y output; dz1y output; dz2y output; z1y input; z2y input
function [dz0y,dz1y,dz2y] = FTDO(p1y,p2y,z0y,z1y,z2y)
r=[24 216 864];
r0=r(1);
r1=r(2);
r2=r(3);
v0=-r0*(abs(z0y-p1y))^(0.8)*sign(z0y-p1y)-r0*(abs(z0y-p1y))^(1.2)*sign(z0y-p1y)+z1y;
dz0y=v0+p2y;
v1=-r1*(abs(z0y-p1y))^(0.6)*sign(z0y-p1y)-r1*(abs(z0y-p1y))^(1.4)*sign(z0y-p1y)+z2y;
dz1y=v1;
dz2y =-r2*(abs(z0y-p1y))^(0.4)*sign(z0y-p1y)-r2*(abs(z0y-p1y))^(1.6)*sign(z0y-p1y);
end

== matlab function paper_Exponential_Predefined_102/MATLAB Function14 ==
  data: t input; dx output; dy output; dz output; delta input; v input; gamma input; psi input
function [dx,dy,dz] = disturbance(t,delta,v,gamma,psi)
fx=-0.0005*abs(v-36)*exp((0.4*v)^0.5)+0.2*sin(psi);
fy=-0.0004*abs(v-30)*exp((0.3*v)^0.5)+0.2*cos(psi);
fz=-0.004*v^(0.5)*sin(3*gamma);
% fx=0;
% fy=0;
% fz=0;
if 0<t && t<10
    wx = 1*sin(t)+delta;
else
    wx=0;
end
if 5<t && t<15
    wy = 2*sin(2*t)-cos(3*t)+delta;
else
    wy=0;
end
if 0<t && t<20
    wz = 0.5*sin(t)+delta;
else
    wz = 0;
end

dx=fx+wx;
dy=fy+wy;
dz=fz+wz;

end

== matlab function paper_Exponential_Predefined_102/MATLAB Function15 ==
  data: p1z input; p2z input; z0z input; dz0z output; dz1z output; dz2z output; z1z input; z2z input
function [dz0z,dz1z,dz2z] = FTDO(p1z,p2z,z0z,z1z,z2z)
r=[24 216 864];
r0=r(1);
r1=r(2);
r2=r(3);
v0=-r0*(abs(z0z-p1z))^(0.8)*sign(z0z-p1z)-r0*(abs(z0z-p1z))^(1.2)*sign(z0z-p1z)+z1z;
dz0z=v0+p2z;
v1=-r1*(abs(z0z-p1z))^(0.6)*sign(z0z-p1z)-r1*(abs(z0z-p1z))^(1.4)*sign(z0z-p1z)+z2z;
dz1z=v1;
dz2z =-r2*(abs(z0z-p1z))^(0.4)*sign(z0z-p1z)-r2*(abs(z0z-p1z))^(1.6)*sign(z0z-p1z);
end

== matlab function paper_Exponential_Predefined_102/MATLAB Function16 ==
  data: p1x input; p2x input; z0x input; dz0x output; dz1x output; dz2x output; z1x input; z2x input
function [dz0x,dz1x,dz2x] = FTDO(p1x,p2x,z0x,z1x,z2x)
r=[24 216 864];%parameters of FTDO
r0=r(1);
r1=r(2);
r2=r(3);
v0=-r0*(abs(z0x-p1x))^(0.8)*sign(z0x-p1x)-r0*(abs(z0x-p1x))^(1.2)*sign(z0x-p1x)+z1x;
dz0x=v0+p2x;
v1=-r1*(abs(z0x-p1x))^(0.6)*sign(z0x-p1x)-r1*(abs(z0x-p1x))^(1.4)*sign(z0x-p1x)+z2x;
dz1x=v1;
dz2x =-r2*(abs(z0x-p1x))^(0.4)*sign(z0x-p1x)-r2*(abs(z0x-p1x))^(1.6)*sign(z0x-p1x);
end

== matlab function paper_Exponential_Predefined_102/X_dot4 ==
  data: vr input; psi_r input; gamma_r input; psi input; gamma input; v input; s1 output; s2 output; s3 output; xr_dot output; yr_dot output; zr_dot output; wx input; wy input; wz input
function [s1,s2,s3,xr_dot,yr_dot,zr_dot] = fcn(vr,psi_r,gamma_r,psi,gamma,v,wx,wy,wz)
wx=0;
wy=0;
wz=0;
s1 = v*cos(psi)*cos(gamma)+wx;
s2 = v*sin(psi)*cos(gamma)+wy;
s3 = v*sin(gamma)+wz;
xr_dot = vr*cos(psi_r)*cos(gamma_r);
yr_dot = vr*sin(psi_r)*cos(gamma_r);
zr_dot = vr*sin(gamma_r);
end

== matlab function paper_Exponential_Predefined_102/control input 4 ==
  data: a_xr input; a_yr input; a_zr input; psi input; gamma input; u1_omiga_psi output; u2_omiga_gamma output; u3_a output; v input; nta_1 input; nta_2 input; nta_3 input
function [u1_omiga_psi,u2_omiga_gamma,u3_a] = fcn(a_xr,a_yr,a_zr,psi,gamma,v,nta_1,nta_2,nta_3)
A = [-a_xr;-a_yr;-a_zr];
B = [-v*sin(psi)*cos(gamma) -v*cos(psi)*sin(gamma) cos(psi)*cos(gamma); 
    v*cos(psi)*cos(gamma) -v*sin(psi)*sin(gamma) sin(psi)*cos(gamma);
    0                        v*cos(gamma)               sin(gamma)];
nta = [nta_1 ; nta_2;nta_3];
U = -inv(B)*(A - nta);
U11=U(1,1); 
U21=U(2,1);
U31=U(3,1);
% 

u1_omiga_psi = U11 ;
u2_omiga_gamma = U21;
u3_a =U31 ;






end

== matlab function paper_Exponential_Predefined_102/f,df4 ==
  data: dx input; x input; dy input; y input; dz input; z input; dxr input; xr input; dyr input; yr input; dzr input; zr input; p1x output; p1y output; p1z output; p2x output; p2y output; p2z output; wx input; wy input; wz input; s1 output; s2 output; s3 output
 function [p1x,p1y,p1z,p2x,p2y,p2z,s1,s2,s3] = fcn(dx,x,dy,y,dz,z,dxr,xr,dyr,yr,dzr,zr,wx,wy,wz)
wx=0;
wy=0;
wz=0;
p1x = x - xr;
p1y = y - yr;
p1z = z - zr;
s1 = dx - dxr ;
s2 = dy - dyr ;
s3 = dz - dzr ;
p2x = dx - dxr-wx ;
p2y = dy - dyr-wy ;
p2z = dz - dzr-wz ;
end

== matlab function paper_Exponential_Predefined_102/u_1a4 ==
  data: u input; u_1a output
function u_1a  = fcn(u)

u_max=1;

u_1a=u_max*erf((pi^(0.5)*u)/(2*u_max));


 end

== matlab function paper_Exponential_Predefined_102/u_2a4 ==
  data: u input; u_2a output
function u_2a  = fcn(u)

u_max=1;

u_2a=u_max*erf((pi^(0.5)*u)/(2*u_max));


 end

== matlab function paper_Exponential_Predefined_102/u_3a4 ==
  data: u input; u_3a output
function u_3a  = fcn(u)

u_max=10;
v_max=15;
% u_3a=u;
u_3a=u_max*erf((pi^(0.5)*u)/(2*u_max));
% q_v=erf((pi^(0.5)*(v-25))/(2*v_max));
% % u_3a=q_u*(1-abs(q_v));
% if v>=40 & u>0
%     u_3a=0;
% elseif v<=10 & u<0
%     u_3a=0;
% else
%     u_3a=u_max*erf((pi^(0.5)*u)/(2*u_max));
    
 end

== matlab function paper_Exponential_Predefined_102/yuding_zhishu4 ==
  data: t input; nta_1 output; t_f input; bta1 input; bta2 input; k1 input; k2 input; p1x input; p1y input; p1z input; p2x input; p2y input; p2z input; z2x input; z2y input; z2z input; nta_2 output; nta_3 output
function [nta_1,nta_2,nta_3] = yuding(t,t_f,bta1,bta2,k1,k2,p1x,p1y,p1z,p2x,p2y,p2z,z2x,z2y,z2z)
z2x=0;
z2y=0;
z2z=0;
x2d=-k1*p1x;
y2d=-k1*p1y;
z2d=-k1*p1z;
sigama2x=p2x-x2d;
sigama2y=p2y-y2d;
sigama2z=p2z-z2d;

nta_1=-p1x+k1-k2*sigama2x;

nta_2=-p1y+k1-k2*sigama2y;

nta_3=-p1z+k1-k2*sigama2z;

   
end

== matlab function paper_Exponential_Predefined_102/ a^r5 ==
  data: ar input; vr input; a_xr output; a_yr output; omiga_psi_r input; psi_r input; omiga_gamma_r input; a_zr output; gamma_r input
function [a_xr,a_yr,a_zr] = fcn(ar,vr,omiga_psi_r,psi_r,omiga_gamma_r,gamma_r)
a_xr = -vr*sin(psi_r)*cos(gamma_r)*omiga_psi_r-vr*cos(psi_r)*sin(gamma_r)*omiga_gamma_r+cos(psi_r)*cos(gamma_r)*ar;
a_yr = vr*cos(psi_r)*cos(gamma_r)*omiga_psi_r-vr*sin(psi_r)*sin(gamma_r)*omiga_gamma_r+ sin(psi_r)*cos(gamma_r)*ar;
a_zr = vr*cos(gamma_r)*omiga_gamma_r + sin(gamma_r)*ar;
end

== matlab function paper_Exponential_Predefined_102/MATLAB Function17 ==
  data: t input; dx output; dy output; dz output; delta input; v input; gamma input; psi input
function [dx,dy,dz] = disturbance(t,delta,v,gamma,psi)
fx=-0.0005*abs(v-36)*exp((0.4*v)^0.5)+0.2*sin(psi);
fy=-0.0004*abs(v-30)*exp((0.3*v)^0.5)+0.2*cos(psi);
fz=-0.004*v^(0.5)*sin(3*gamma);
% fx=0;
% fy=0;
% fz=0;
if 0<t && t<10
    wx = 1*sin(t)+delta;
else
    wx=0;
end
if 5<t && t<15
    wy = 2*sin(2*t)-cos(3*t)+delta;
else
    wy=0;
end
if 0<t && t<20
    wz = 0.5*sin(t)+delta;
else
    wz = 0;
end

dx=fx+wx;
dy=fy+wy;
dz=fz+wz;

end

== matlab function paper_Exponential_Predefined_102/MATLAB Function18 ==
  data: p1z input; p2z input; z0z input; dz0z output; dz1z output; dz2z output; z1z input; z2z input
function [dz0z,dz1z,dz2z] = FTDO(p1z,p2z,z0z,z1z,z2z)
r=[24 216 864];
r0=r(1);
r1=r(2);
r2=r(3);
v0=-r0*(abs(z0z-p1z))^(0.8)*sign(z0z-p1z)-r0*(abs(z0z-p1z))^(1.2)*sign(z0z-p1z)+z1z;
dz0z=v0+p2z;
v1=-r1*(abs(z0z-p1z))^(0.6)*sign(z0z-p1z)-r1*(abs(z0z-p1z))^(1.4)*sign(z0z-p1z)+z2z;
dz1z=v1;
dz2z =-r2*(abs(z0z-p1z))^(0.4)*sign(z0z-p1z)-r2*(abs(z0z-p1z))^(1.6)*sign(z0z-p1z);
end

== matlab function paper_Exponential_Predefined_102/MATLAB Function19 ==
  data: p1x input; p2x input; z0x input; dz0x output; dz1x output; dz2x output; z1x input; z2x input
function [dz0x,dz1x,dz2x] = FTDO(p1x,p2x,z0x,z1x,z2x)
r=[24 216 864];
r0=r(1);
r1=r(2);
r2=r(3);
v0=-r0*(abs(z0x-p1x))^(0.8)*sign(z0x-p1x)-r0*(abs(z0x-p1x))^(1.2)*sign(z0x-p1x)+z1x;
dz0x=v0+p2x;
% dz0x=v0;
v1=-r1*(abs(z0x-p1x))^(0.6)*sign(z0x-p1x)-r1*(abs(z0x-p1x))^(1.4)*sign(z0x-p1x)+z2x;
dz1x=v1;
dz2x =-r2*(abs(z0x-p1x))^(0.4)*sign(z0x-p1x)-r2*(abs(z0x-p1x))^(1.6)*sign(z0x-p1x);
end

== matlab function paper_Exponential_Predefined_102/MATLAB Function20 ==
  data: p1y input; p2y input; z0y input; dz0y output; dz1y output; dz2y output; z1y input; z2y input
function [dz0y,dz1y,dz2y] = FTDO(p1y,p2y,z0y,z1y,z2y)
r=[24 216 864];
r0=r(1);
r1=r(2);
r2=r(3);
v0=-r0*(abs(z0y-p1y))^(0.8)*sign(z0y-p1y)-r0*(abs(z0y-p1y))^(1.2)*sign(z0y-p1y)+z1y;
dz0y=v0+p2y;
v1=-r1*(abs(z0y-p1y))^(0.6)*sign(z0y-p1y)-r1*(abs(z0y-p1y))^(1.4)*sign(z0y-p1y)+z2y;
dz1y=v1;
dz2y =-r2*(abs(z0y-p1y))^(0.4)*sign(z0y-p1y)-r2*(abs(z0y-p1y))^(1.6)*sign(z0y-p1y);
end

== matlab function paper_Exponential_Predefined_102/X_dot5 ==
  data: vr input; psi_r input; gamma_r input; psi input; gamma input; v input; s1 output; s2 output; s3 output; xr_dot output; yr_dot output; zr_dot output; wx input; wy input; wz input
function [s1,s2,s3,xr_dot,yr_dot,zr_dot] = fcn(vr,psi_r,gamma_r,psi,gamma,v,wx,wy,wz)
% wx=0;
% wy=0;
% wz=0;
s1 = v*cos(psi)*cos(gamma)+wx;
s2 = v*sin(psi)*cos(gamma)+wy;
s3 = v*sin(gamma)+wz;
xr_dot = vr*cos(psi_r)*cos(gamma_r);
yr_dot = vr*sin(psi_r)*cos(gamma_r);
zr_dot = vr*sin(gamma_r);
end
